simulink model "OMSv1_5_lfd"  (Simulink 7.0)
settings: Solver=ode4  SolverMode=SingleTasking  StartTime=0.0  StopTime=5  FixedStep=0.001  MaxStep=0.001  RelTol=1e-3  AbsTol=1e-3
undefined symbols (not defined in the file): alexlaw, bs_onoff, bs_scale, bsfsacrit, bsfsvcrit, cnsgain, fs_onoff, fs_scale, fsdelaycalc, ltdrk, mdlparamlist, phasicgain, pmcgain, pmctau2, pmctau3, saccsw, spgain, tonicgain, tvrD, tvrN
(part 2 of 11)

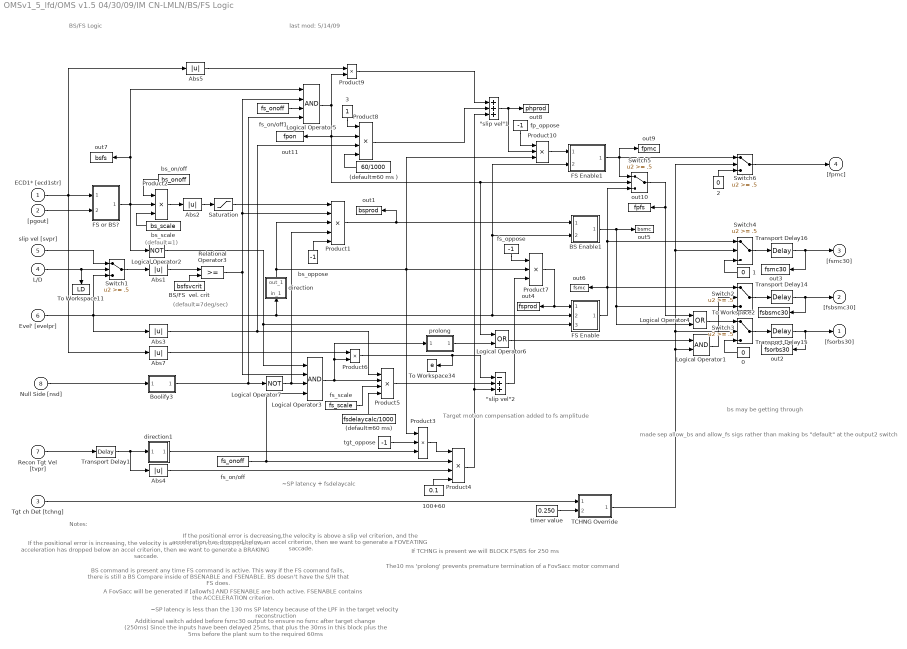
== system OMSv1_5_lfd/OMS v1.5 04/30/09/IM CN-LMLN/BS/FS Logic ==
  note: BS/FS Logic
  note: If the positional error is increasing, the velocity
      |  is above a slip vel criterion, and the acceleration
      | has dropped below an accel criterion, then we
      | want to generate a BRAKING saccade.
  note: If the positional error is decreasing,the velocity
      | is above a slip vel criterion, and the acceleration
      | has dropped below an accel criterion, then we
      | want to generate a FOVEATING saccade.
  note: last mod:
      | 5/14/09
  note: (default=7deg/sec)
  note: (default=1)
  note: If TCHNG is present we will BLOCK
      | FS/BS for 250 ms
  note: BS command is present any time FS command is active.  This way if the FS coomand fails, there is still a BS
      | Compare inside of BSENABLE and FSENABLE.  BS doesn't have the S/H that FS does.
  note: A FovSacc will be generated if [allowfs] AND FSENABLE are both active. FSENABLE contains the ACCELERATION criterion.
  note: Notes:
  note: The10 ms 'prolong' prevents premature
      | termination of a FovSacc motor command
  note: made sep allow_bs and allow_fs
      | sigs rather than making bs "default"
      | at the output2 switch
  note: bs may be getting through
  note: ~SP latency + fsdelaycalc
  note: Target motion compensation
      | added to fs amplitude
  note: ~SP latency is less than the 130 ms SP latency because of the LPF in the target velocity reconstruction
  note: Additional switch added before fsmc30 output to ensure no fsmc after target change (250ms)
      | Since the inputs have been delayed 25ms, that plus the 30ms in this block plus the 5ms before the plant sum to the required 60ms
  ECD1* [ecd1str] : Inport  OutDataType=sfix(16)  OutScaling=2^0
  "[pgout]" : Inport  Port=2  OutDataType=sfix(16)  OutScaling=2^0
  Tgt ch Det [tchng] : Inport  Port=3  OutDataType=sfix(16)  OutScaling=2^0
  L/D : Inport  Port=4  OutDataType=sfix(16)  OutScaling=2^0
  slip vel [svpr] : Inport  Port=5  OutDataType=sfix(16)  OutScaling=2^0
  Evel' [evelpr] : Inport  Port=6  OutDataType=sfix(16)  OutScaling=2^0
  Recon Tgt Vel [tvpr] : Inport  Port=7  OutDataType=sfix(16)  OutScaling=2^0
  Null Side [nsd] : Inport  Port=8  OutDataType=sfix(16)  OutScaling=2^0
  "\"slip vel\"1" : Sum  Inputs=+++  OutDataType=sfix(16)  OutScaling=2^0  SaturateOnIntegerOverflow=on  InputSameDT=on
  "\"slip vel\"2" : Sum  Inputs=-++  OutDataType=sfix(16)  OutScaling=2^0  SaturateOnIntegerOverflow=on  InputSameDT=on
  (default=60 ms ) : Constant  Orientation=left  Value=60/1000  OutDataType=sfix(16)  OutScaling=2^0
  (default=60 ms) : Constant  Orientation=up  Value=fsdelaycalc/1000  OutDataType=sfix(16)  OutScaling=2^0
  0 : Constant  Orientation=left  Value=0  OutDataType=sfix(16)  OutScaling=2^0
  1 : Constant  Orientation=left  Value=0  OutDataType=sfix(16)  OutScaling=2^0
  100+60 : Constant  Orientation=up  Value=0.1  OutDataType=sfix(16)  OutScaling=2^0
  2 : Constant  Orientation=up  Value=0  OutDataType=sfix(16)  OutScaling=2^0
  3 : Constant  Orientation=down  OutDataType=sfix(16)  OutScaling=2^0
  Abs{1..5,7} (6 alike) : Abs  SaturateOnIntegerOverflow=on
  BS Enable1 : Subsystem
      mask Display: disp('BS\nEnab')
  BS/FS  vel. crit : Constant  Orientation=up  Value=bsfsvcrit  OutDataType=sfix(16)  OutScaling=2^0
  Boolify3 : Subsystem
      mask Display: disp('Boolify')
  FS Enable : Subsystem
      mask Display: disp('FS\nEnab')
  FS Enable1 : Subsystem
      mask Display: disp('Fast Phase\nEnab')
  FS or BS? : Subsystem
      mask Display: disp('BS=1\nFS=0')
  Logical Operator1 : Logic
  Logical Operator2 : Logic  Operator=NOT  Inputs=1
  Logical Operator3 : Logic  Inputs=4
  Logical Operator4 : Logic  Operator=OR
  Logical Operator5 : Logic  Inputs=4
  Logical Operator6 : Logic  Operator=OR
  Logical Operator7 : Logic  Operator=NOT  Inputs=1
  Product1 : Product  Inputs=5  OutDataType=sfix(16)  OutScaling=2^0  SaturateOnIntegerOverflow=on  RndMeth=Zero  InputSameDT=on
  Product{2..3,7,10} (4 alike) : Product  Inputs=3  OutDataType=sfix(16)  OutScaling=2^0  SaturateOnIntegerOverflow=on  RndMeth=Zero  InputSameDT=on
  Product4 : Product  Inputs=4  OutDataType=sfix(16)  OutScaling=2^0  SaturateOnIntegerOverflow=on  RndMeth=Zero  InputSameDT=on
  Product5 : Product  Inputs=4  OutDataType=sfix(16)  OutScaling=2^0  SaturateOnIntegerOverflow=on  RndMeth=Zero  InputSameDT=on
  Product6 : Product  OutDataType=sfix(16)  OutScaling=2^0  SaturateOnIntegerOverflow=on  RndMeth=Zero  InputSameDT=on
  Product8 : Product  Inputs=4  OutDataType=sfix(16)  OutScaling=2^0  SaturateOnIntegerOverflow=on  RndMeth=Zero  InputSameDT=on
  Product9 : Product  OutDataType=sfix(16)  OutScaling=2^0  SaturateOnIntegerOverflow=on  RndMeth=Zero  InputSameDT=on
  Relational Operator3 : RelationalOperator  InputSameDT=on
  Saturation : Saturate  UpperLimit=2  LowerLimit=0
  Switch{1..6} (6 alike) : Switch  Threshold=.5  SaturateOnIntegerOverflow=on  InputSameDT=on
  TCHNG Override : Subsystem
      mask Display: disp('TCHNG\nOverride')
  To Workspace11 : ToWorkspace  VariableName=LD  SaveFormat=Array
      settings: Orientation=down  MaxDataPoints=10000
  To Workspace2 : ToWorkspace  VariableName=fsbsmc30  SaveFormat=Array
      settings: MaxDataPoints=10000
  To Workspace34 : ToWorkspace  VariableName=e  SaveFormat=Array
      settings: MaxDataPoints=10000
  Transport Delay1 : TransportDelay  DelayTime=0.05
      mask Display: disp('50ms')
  Transport Delay14 : TransportDelay  DelayTime=0.03
      mask Display: disp('30ms')
  Transport Delay15 : TransportDelay  DelayTime=0.03
      mask Display: disp('30ms')
  Transport Delay16 : TransportDelay  DelayTime=0.03
      mask Display: disp('30ms')
  bs_on/off : Constant  Orientation=left  Value=bs_onoff  OutDataType=sfix(16)  OutScaling=2^0
  bs_oppose : Constant  Orientation=up  Value=-1  OutDataType=sfix(16)  OutScaling=2^0
  bs_scale : Constant  Orientation=left  Value=bs_scale  OutDataType=sfix(16)  OutScaling=2^0
  direction : Subsystem  Orientation=up
      mask Type: Sign
      mask Description: y = sign(x)
      mask Help: Sign Function:\n\t\t\ty = 1 if x > 0\n\t\t\ty = 0 if x = 0\n\t\t\ty = -1 if x < 0
      mask Display: plot(-50,-50,50,50,[-50,50],[0,0],[0,0],[-50,50],[-40,0],[-30,-30],[0,40],[30,30])
  direction1 : Subsystem
      mask Type: Sign
      mask Description: y = sign(x)
      mask Help: Sign Function:\n\t\t\ty = 1 if x > 0\n\t\t\ty = 0 if x = 0\n\t\t\ty = -1 if x < 0
      mask Display: plot(-50,-50,50,50,[-50,50],[0,0],[0,0],[-50,50],[-40,0],[-30,-30],[0,40],[30,30])
  fp_oppose : Constant  Orientation=down  Value=-1  OutDataType=sfix(16)  OutScaling=2^0
  fs_on/off : Constant  Value=fs_onoff  OutDataType=sfix(16)  OutScaling=2^0
  fs_on/off1 : Constant  Value=fs_onoff  OutDataType=sfix(16)  OutScaling=2^0
  fs_oppose : Constant  Orientation=down  Value=-1  OutDataType=sfix(16)  OutScaling=2^0
  fs_scale : Constant  Value=fs_scale  OutDataType=sfix(16)  OutScaling=2^0
  out1 : ToWorkspace  VariableName=bsprod  SaveFormat=Array
      settings: MaxDataPoints=100000
  out10 : ToWorkspace  VariableName=fpfs  SaveFormat=Array
      settings: MaxDataPoints=100000
  out11 : ToWorkspace  VariableName=fpon  SaveFormat=Array
      settings: MaxDataPoints=100000
  out2 : ToWorkspace  VariableName=fsorbs30  SaveFormat=Array
      settings: MaxDataPoints=100000
  out3 : ToWorkspace  VariableName=fsmc30  SaveFormat=Array
      settings: MaxDataPoints=100000
  out4 : ToWorkspace  VariableName=fsprod  SaveFormat=Array
      settings: MaxDataPoints=100000
  out5 : ToWorkspace  VariableName=bsmc  SaveFormat=Array
      settings: MaxDataPoints=100000
  out6 : ToWorkspace  VariableName=fsmc  SaveFormat=Array
      settings: MaxDataPoints=100000
  out7 : ToWorkspace  VariableName=bsfs  SaveFormat=Array
      settings: MaxDataPoints=100000
  out8 : ToWorkspace  VariableName=phprod  SaveFormat=Array
      settings: MaxDataPoints=100000
  out9 : ToWorkspace  VariableName=fpmc  SaveFormat=Array
      settings: MaxDataPoints=100000
  prolong : Subsystem  mask{prolong=1}
      mask prompts: prolong "Prolong pulse by?  (msec)"
      mask Display: disp('prolong')
  tgt_oppose : Constant  Value=-1  OutDataType=sfix(16)  OutScaling=2^0
  timer value : Constant  Value=0.250  OutDataType=sfix(16)  OutScaling=2^0
  "[fsorbs30]" : Outport  OutDataType=sfix(16)  OutScaling=2^0  InitialOutput=0
  "[fsbsmc30]" : Outport  Port=2  OutDataType=sfix(16)  OutScaling=2^0  InitialOutput=0
  "[fsmc30]" : Outport  Port=3  OutDataType=sfix(16)  OutScaling=2^0  InitialOutput=0
  "[fpmc]" : Outport  Port=4  OutDataType=sfix(16)  OutScaling=2^0  InitialOutput=0
  wires:
  Abs2/1 -> Saturation/1
  FS or BS?/1(BS=1 FS=0) -> Product2/2, Logical Operator2/1, Logical Operator5/1, out7/1
  bs_on/off/1 -> Product2/1
  bs_scale/1 -> Product2/3
  slip vel [svpr]/1 -> Switch1/1
  Switch1/1 -> Abs1/1
  Evel' [evelpr]/1 -> Switch1/3, direction/1(in_1), FS Enable/2("[evelpr]"), BS Enable1/2("[evelpr]"), FS Enable1/2("[evelpr]"), Abs3/1
  Relational Operator3/1 -> Logical Operator3/2, Product1/2, Logical Operator5/2
  "[pgout]"/1 -> FS or BS?/2(pgout)
  ECD1* [ecd1str]/1 -> Abs5/1, FS or BS?/1(pos error [ecd1str]), Abs7/1
  BS/FS  vel. crit/1 -> Relational Operator3/2
  Abs1/1 -> Relational Operator3/1
  direction/1(out_1) -> Product1/3, Product7/2, Product10/3, Product3/1
  (default=60 ms)/1 -> Product5/4
  Abs3/1 -> Product5/1, Product8/3
  Logical Operator3/1 -> Product5/2, Product6/2, prolong/1(value(in))
  fs_oppose/1 -> Product7/1
  Abs7/1 -> Product6/1
  FS Enable/1("[fsmc]") -> Switch2/1, out6/1, Switch4/1, Switch5/3
  Switch2/1 -> Transport Delay14/1
  fs_scale/1 -> Product5/3
  Tgt ch Det [tchng]/1 -> TCHNG Override/1("[tchng]")
  timer value/1 -> TCHNG Override/2(timer dur)
  Transport Delay14/1 -> "[fsbsmc30]"/1, To Workspace2/1
  TCHNG Override/1(tchng sw) -> Switch4/2, Switch6/2, Switch3/2, Logical Operator1/2
  Transport Delay16/1 -> "[fsmc30]"/1, out3/1
  Product2/1 -> Abs2/1
  Saturation/1 -> Product1/1
  Product5/1 -> "\"slip vel\"2"/2
  Product7/1 -> FS Enable/1(fsprod), out4/1
  Product1/1 -> out1/1, BS Enable1/1(bsprod)
  BS Enable1/1("[bsmc]") -> out5/1, Switch2/3, Logical Operator4/2
  Logical Operator4/1 -> Switch3/1
  Switch3/1 -> Transport Delay15/1
  L/D/1 -> Switch1/2, To Workspace11/1
  Recon Tgt Vel [tvpr]/1 -> Transport Delay1/1
  Product3/1 -> Product4/1
  100+60/1 -> Product4/4
  direction1/1(out_1) -> Product3/3
  Abs4/1 -> Product4/3
  Product4/1 -> "\"slip vel\"2"/3, "\"slip vel\"1"/3
  "\"slip vel\"2"/1 -> Product7/3
  0/1 -> Switch3/3
  Logical Operator1/1 -> Switch2/2
  1/1 -> Switch4/3
  Switch4/1 -> Transport Delay16/1
  Transport Delay15/1 -> "[fsorbs30]"/1, out2/1
  Logical Operator2/1 -> Logical Operator3/1, FS Enable/3(fsbs?)
  Transport Delay1/1 -> direction1/1(in_1), Abs4/1
  Boolify3/1(Out1) -> Logical Operator7/1, Logical Operator5/4
  Null Side [nsd]/1 -> Boolify3/1(In1)
  fs_on/off/1 -> Product4/2, Logical Operator3/4
  Logical Operator7/1 -> Logical Operator3/3, Product1/4
  Logical Operator5/1 -> Product9/2, Product8/2, out11/1, Switch5/2, Logical Operator6/1
  (default=60 ms )/1 -> Product8/4
  Product8/1 -> "\"slip vel\"1"/2
  Product9/1 -> "\"slip vel\"1"/1
  "\"slip vel\"1"/1 -> out8/1, Product10/2
  fp_oppose/1 -> Product10/1
  Product10/1 -> FS Enable1/1(fsprod)
  FS Enable1/1("[fsmc]") -> Switch5/1, out9/1, Switch6/1
  2/1 -> Switch6/3
  Switch6/1 -> "[fpmc]"/1
  fs_on/off1/1 -> Logical Operator5/3
  Abs5/1 -> Product9/1
  3/1 -> Product8/1
  bs_oppose/1 -> Product1/5
  tgt_oppose/1 -> Product3/2
  Switch5/1 -> Logical Operator4/1, out10/1
  Logical Operator6/1 -> Logical Operator1/1
  Product6/1 -> "\"slip vel\"2"/1, To Workspace34/1
  prolong/1(value(out)) -> Logical Operator6/2

== system OMSv1_5_lfd/OMS v1.5 04/30/09/IM CN-LMLN/MdlPlnt+2 ==
  note: Plant Model+
  note: last mod:
      | 06/13/07
  note: fast
  note: slow
  "[eposspf]" : Inport  OutDataType=sfix(16)  OutScaling=2^0
  "[pgout]" : Inport  Port=2  OutDataType=sfix(16)  OutScaling=2^0
  "[epossps]" : Inport  Port=3  OutDataType=sfix(16)  OutScaling=2^0
  Derivative : Derivative
      mask Display: disp('s')
  NI Real2 : Subsystem
      mask Display: disp('Plant')
  OMN1 : Subsystem
      mask Display: disp('Slow\nOMN')
  OMN3 : Subsystem
      mask Display: disp('Fast\nOMN')
  To Workspace13 : ToWorkspace  VariableName=ecpy80  SaveFormat=Array
      settings: MaxDataPoints=10000
  To Workspace28 : ToWorkspace  VariableName=imvel  SaveFormat=Array
      settings: Orientation=down  MaxDataPoints=10000
      mask Type: imsw1in
  Transport Delay1 : TransportDelay  DelayTime=0.005
      mask Display: disp('5ms')
  Transport Delay12 : TransportDelay  DelayTime=0.075
      mask Display: disp('75ms')
  Transport Delay2 : TransportDelay  DelayTime=0.075
      mask Display: disp('75ms')
  Transport Delay3 : TransportDelay  DelayTime=0.005
      mask Display: disp('5ms')
  "[ecpy80]" : Outport  OutDataType=sfix(16)  OutScaling=2^0  InitialOutput=0
  "[imvel]" : Outport  Port=2  OutDataType=sfix(16)  OutScaling=2^0  InitialOutput=0
  wires:
  Derivative/1 -> Transport Delay2/1
  Transport Delay12/1 -> "[ecpy80]"/1, To Workspace13/1
  OMN3/1("[psout]") -> Transport Delay3/1
  Transport Delay1/1 -> NI Real2/2(slow components)
  OMN1/1("[psout]") -> Transport Delay1/1
  Transport Delay3/1 -> NI Real2/1(fast components)
  NI Real2/1(ecpyy) -> Derivative/1, Transport Delay12/1
  "[pgout]"/1 -> OMN3/2("[pgout]")
  "[eposspf]"/1 -> OMN3/1("[epossp]")
  Transport Delay2/1 -> "[imvel]"/1, To Workspace28/1
  "[epossps]"/1 -> OMN1/1("[epossp]")

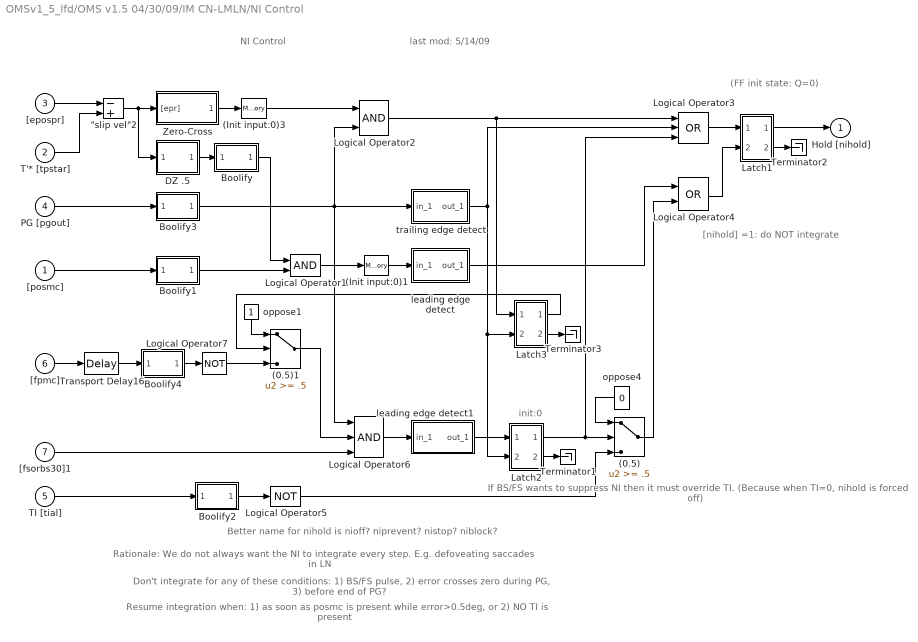
== system OMSv1_5_lfd/OMS v1.5 04/30/09/IM CN-LMLN/NI Control ==
  note: (FF init state: Q=0)
  note: NI Control
  note: If BS/FS wants to suppress NI
      | then it must override TI. (Because
      | when TI=0, nihold is forced off)
  note: last mod:
      | 5/14/09
  note: Rationale: We do not always want the NI to integrate every step. E.g. defoveating saccades in LN
  note: Don't integrate for any of these conditions: 1) BS/FS pulse, 2) error crosses zero during PG, 3) before end of PG?
  note: [nihold] =1: do NOT integrate
  note: init:0
  note: Better name for nihold is nioff? niprevent? nistop? niblock?
  note: Resume integration when: 1) as soon as posmc is present while error>0.5deg, or 2) NO TI is present
  "[posmc]" : Inport  OutDataType=sfix(16)  OutScaling=2^0
  T'* [tpstar] : Inport  Port=2  OutDataType=sfix(16)  OutScaling=2^0
  "[epospr]" : Inport  Port=3  OutDataType=sfix(16)  OutScaling=2^0
  PG [pgout] : Inport  Port=4  OutDataType=sfix(16)  OutScaling=2^0
  TI [tial] : Inport  Port=5  OutDataType=sfix(16)  OutScaling=2^0
  "[fpmc]" : Inport  Port=6  OutDataType=sfix(16)  OutScaling=2^0
  "[fsorbs30]1" : Inport  Port=7  OutDataType=sfix(16)  OutScaling=2^0
  "\"slip vel\"2" : Sum  Inputs=-+  OutDataType=sfix(16)  OutScaling=2^0  SaturateOnIntegerOverflow=on  InputSameDT=on
  (0.5) : Switch  Threshold=.5  SaturateOnIntegerOverflow=on  InputSameDT=on
  (0.5)1 : Switch  Threshold=.5  SaturateOnIntegerOverflow=on  InputSameDT=on
  (Init input:0)1 : Memory
  (Init input:0)3 : Memory
  Boolify : Subsystem
      mask Display: disp('Boolify')
  Boolify1 : Subsystem
      mask Display: disp('Boolify')
  Boolify2 : Subsystem
      mask Display: disp('Boolify')
  Boolify3 : Subsystem
      mask Display: disp('Boolify')
  Boolify4 : Subsystem
      mask Display: disp('Boolify')
  DZ .5 : Subsystem
      mask Display: disp('Dead\nZone')
  Latch1 : Subsystem  mask(Latch){@1=0}
      mask prompts: @1 "Initial State for Output "Q":"
      mask help: Latch
      mask init:
      | ini=(@1~=0);
      mask Help: Latches the S input.  When S (set) is one, the Q output  becomes one.  The output remains one until the R (reset) input becomes one, forcing the output to zero.  If both R and S are one, the latch will be in an undefined state.
      mask Display: disp('S   Q\n\nR  !Q')
  Latch2 : Subsystem  mask(Latch){@1=0}
      mask prompts: @1 "Initial State for Output "Q":"
      mask help: Latch
      mask init:
      | ini=(@1~=0);
      mask Help: Latches the S input.  When S (set) is one, the Q output  becomes one.  The output remains one until the R (reset) input becomes one, forcing the output to zero.  If both R and S are one, the latch will be in an undefined state.
      mask Display: disp('S   Q\n\nR  !Q')
  Latch3 : Subsystem  mask(Latch){@1=0}
      mask prompts: @1 "Initial State for Output "Q":"
      mask help: Latch
      mask init:
      | ini=(@1~=0);
      mask Help: Latches the S input.  When S (set) is one, the Q output  becomes one.  The output remains one until the R (reset) input becomes one, forcing the output to zero.  If both R and S are one, the latch will be in an undefined state.
      mask Display: disp('S   Q\n\nR  !Q')
  Logical Operator1 : Logic
  Logical Operator2 : Logic
  Logical Operator3 : Logic  Operator=OR  Inputs=3
  Logical Operator4 : Logic  Operator=OR
  Logical Operator5 : Logic  Operator=NOT  Inputs=1
  Logical Operator6 : Logic  Inputs=3
  Logical Operator7 : Logic  Operator=NOT  Inputs=1
  Terminator1 : Terminator
  Terminator2 : Terminator
  Terminator3 : Terminator
  Transport Delay16 : TransportDelay  DelayTime=0.03
      mask Display: disp('30ms')
  Zero-Cross : Subsystem
      mask Display: disp('Zero-Cross\nDetect')
  leading edge detect : Subsystem
      mask Display: disp('Leading\nEdge Det')
  leading edge detect1 : Subsystem
      mask Display: disp('Leading\nEdge Det')
  oppose1 : Constant  Orientation=down  OutDataType=sfix(16)  OutScaling=2^0
  oppose4 : Constant  Orientation=left  Value=0  OutDataType=sfix(16)  OutScaling=2^0
  trailing edge detect : Subsystem
      mask Display: disp('Trailing\nEdge Det')
  Hold [nihold] : Outport  OutDataType=sfix(16)  OutScaling=2^0  InitialOutput=0
  wires:
  T'* [tpstar]/1 -> "\"slip vel\"2"/2
  PG [pgout]/1 -> Boolify3/1(In1)
  "[epospr]"/1 -> "\"slip vel\"2"/1
  Latch1/1(out_1) -> Hold [nihold]/1
  Logical Operator1/1 -> (Init input:0)1/1
  oppose4/1 -> (0.5)/1
  Logical Operator5/1 -> (0.5)/3
  TI [tial]/1 -> Boolify2/1(In1)
  Boolify2/1(Out1) -> Logical Operator5/1
  (0.5)/1 -> Logical Operator4/2
  Boolify3/1(Out1) -> Logical Operator6/1, trailing edge detect/1(in_1), Logical Operator2/2
  trailing edge detect/1(out_1) -> Logical Operator3/2, Latch2/2(in_2), Latch3/2(in_2)
  "[posmc]"/1 -> Boolify1/1(In1)
  "\"slip vel\"2"/1 -> DZ .5/1(in_1), Zero-Cross/1("[epr]")
  Logical Operator2/1 -> Logical Operator3/1, Latch3/1(in_1)
  Logical Operator3/1 -> Latch1/1(in_1)
  Logical Operator4/1 -> Latch1/2(in_2)
  leading edge detect/1(out_1) -> Logical Operator4/1
  Boolify/1(Out1) -> Logical Operator1/1
  DZ .5/1(out_1) -> Boolify/1(In1)
  Boolify1/1(Out1) -> Logical Operator1/2
  Logical Operator6/1 -> leading edge detect1/1(in_1)
  leading edge detect1/1(out_1) -> Latch2/1(in_1)
  Latch2/2(out_2) -> Terminator1/1
  Latch1/2(out_2) -> Terminator2/1
  Zero-Cross/1("[epneq]") -> (Init input:0)3/1
  (Init input:0)3/1 -> Logical Operator2/1
  (Init input:0)1/1 -> leading edge detect/1(in_1)
  "[fsorbs30]1"/1 -> Logical Operator6/3
  Latch3/2(out_2) -> Terminator3/1
  (0.5)1/1 -> Logical Operator6/2
  Latch3/1(out_1) -> (0.5)1/2
  oppose1/1 -> (0.5)1/1
  Transport Delay16/1 -> Boolify4/1(In1)
  Boolify4/1(Out1) -> Logical Operator7/1
  "[fpmc]"/1 -> Transport Delay16/1
  Logical Operator7/1 -> (0.5)1/3
  Latch2/1(out_1) -> (0.5)/2, Logical Operator3/3

== system OMSv1_5_lfd/OMS v1.5 04/30/09/IM CN-LMLN/Sacc Blank ==
  note: Saccade and Post-Saccadic Drift Blanking
  note: (FF init state: Q=1)
  note: "Is RetVel Err increaing?"
  note: really an "enable"
      | signal?
  note: last mod:
      | 02/03/00
  note: [sbsac]  is initially ENABLED, and is DISABLED by  the leading edge of a saccade
      |  (after an 80ms delay).  70 ms later the timer REENABLES [sbsac]
      | (Because of the 80ms delay, actual time of reenable is150 ms after end of PG)
  note: Lower SR latch is SET by [sbsac] going high.  The switch will now pass information
      | about the change in velocity error (whether it is decreasing or increasing).
      | If it is increasing, [sbsp] is 1, and the beginning of this increase sets the switch so
      | that [sbsp] = [sbsac].  If the error is decreasing, then [sbsp] = 0, and should stay 0
      |  for as long as [velerr] is decreasing ***and hasn't crossed zero***
  note: Rationale: We do not want the model to look at the slow phase information that immediately
      | follows a saccade.   We want to disable both the saccadic and SP systems appropriately.
  note: Saccadic:
  note: SP:
  note: (init: Q=0)
  note: "non-decreasing"
  PG [pgout] : Inport  OutDataType=sfix(16)  OutScaling=2^0
  RetVelErr [velerr] : Inport  Port=2  OutDataType=sfix(16)  OutScaling=2^0
  Abs1 : Abs  SaturateOnIntegerOverflow=on
  Latch1 : Subsystem  mask(Latch){@1=1}
      mask prompts: @1 "Initial State for Output "Q":"
      mask help: Latch
      mask init:
      | ini=(@1~=0);
      mask Help: Latches the S input.  When S (set) is one, the Q output  becomes one.  The output remains one until the R (reset) input becomes one, forcing the output to zero.  If both R and S are one, the latch will be in an undefined state.
      mask Display: disp('S   Q\n\nR  !Q')
  Latch2 : Subsystem  mask(Latch){@1=0}
      mask prompts: @1 "Initial State for Output "Q":"
      mask help: Latch
      mask init:
      | ini=(@1~=0);
      mask Help: Latches the S input.  When S (set) is one, the Q output  becomes one.  The output remains one until the R (reset) input becomes one, forcing the output to zero.  If both R and S are one, the latch will be in an undefined state.
      mask Display: disp('S   Q\n\nR  !Q')
  Relational Operator : RelationalOperator  InputSameDT=on
  Switch5 : Switch  Threshold=.5  SaturateOnIntegerOverflow=on  InputSameDT=on
  Terminator : Terminator
  Terminator1 : Terminator
  To Workspace10 : ToWorkspace  VariableName=sbred  SaveFormat=Array
      settings: MaxDataPoints=10000
  To Workspace16 : ToWorkspace  VariableName=sbsac  SaveFormat=Array
      settings: MaxDataPoints=10000
  To Workspace22 : ToWorkspace  VariableName=sbsp  SaveFormat=Array
      settings: MaxDataPoints=10000
  Transport Delay1 : TransportDelay  DelayTime=0.08
      mask Display: disp('80ms')
  event timer1 : Subsystem
      mask Display: disp('Event\nTimer2')
  leading edge detect : Subsystem
      mask Display: disp('Leading\nEdge Det')
  loop breaker : Memory
  rising edge detect : Subsystem  Orientation=left
      mask Display: disp('Rising\nEdge Det')
  rising edge detect1 : Subsystem
      mask Display: disp('Rising\nEdge Det')
  timer value : Constant  Orientation=left  Value=0.07  OutDataType=sfix(16)  OutScaling=2^0
  SacBlnk [sbsac] : Outport  OutDataType=sfix(16)  OutScaling=2^0  InitialOutput=0
  SP S/H [sbsp] : Outport  Port=2  OutDataType=sfix(16)  OutScaling=2^0  InitialOutput=0
  wires:
  leading edge detect/1(out_1) -> Latch1/2(in_2)
  event timer1/1(out_1) -> Latch1/1(in_1)
  loop breaker/1 -> Relational Operator/2
  Abs1/1 -> loop breaker/1, Relational Operator/1
  Relational Operator/1 -> rising edge detect/1(in_1), Switch5/1
  rising edge detect1/1(out_1) -> To Workspace10/1, Latch2/1(in_1)
  RetVelErr [velerr]/1 -> Abs1/1
  PG [pgout]/1 -> Transport Delay1/1
  Transport Delay1/1 -> leading edge detect/1(in_1), event timer1/1(_PG)
  timer value/1 -> event timer1/2(_timer value (port))
  Latch1/1(out_1) -> SacBlnk [sbsac]/1, rising edge detect1/1(in_1), Switch5/3, To Workspace16/1
  rising edge detect/1(out_1) -> Latch2/2(in_2)
  Latch2/1(out_1) -> Switch5/2
  Switch5/1 -> SP S/H [sbsp]/1, To Workspace22/1
  Latch2/2(out_2) -> Terminator/1
  Latch1/2(out_2) -> Terminator1/1

== system OMSv1_5_lfd/OMS v1.5 04/30/09/IM CN-LMLN/Saccade Enable ==
  note: Saccade Enable
  note: last mod:
      | 07/11/07
  note: rfbenctrl
  note: ecenctrl
  note: e'*DZ
  note: for LN: make this
      | (fsorbs OR fphsz)
  note: TIDZ
  Tgt ch Det [tchng] : Inport  OutDataType=sfix(16)  OutScaling=2^0
  "[ecdstrdz]" : Inport  Port=2  OutDataType=sfix(16)  OutScaling=2^0
  "[err50]" : Inport  Port=3  OutDataType=sfix(16)  OutScaling=2^0
  "[pgout]" : Inport  Port=4  OutDataType=sfix(16)  OutScaling=2^0
  "[edot50]" : Inport  Port=5  OutDataType=sfix(16)  OutScaling=2^0
  "[tial]" : Inport  Port=6  OutDataType=sfix(16)  OutScaling=2^0
  "[sbsac]" : Inport  Port=7  OutDataType=sfix(16)  OutScaling=2^0
  "[fsorbs30]" : Inport  Port=8  OutDataType=sfix(16)  OutScaling=2^0
  Enable Control : Subsystem
      mask Display: disp('Enable\nControl')
  LN FPh Gen : Subsystem
      mask Display: disp('DFFPh\nGen')
  Latch1 : Subsystem  mask(Latch){@1=0}
      mask prompts: @1 "Initial State for Output "Q":"
      mask help: Latch
      mask init:
      | ini=(@1~=0);
      mask Help: Latches the S input.  When S (set) is one, the Q output  becomes one.  The output remains one until the R (reset) input becomes one, forcing the output to zero.  If both R and S are one, the latch will be in an undefined state.
      mask Display: disp('S   Q\n\nR  !Q')
  Logical Operator2 : Logic  Operator=NOT  Inputs=1
  Logical Operator3 : Logic
  Ret FB sample : Subsystem
      mask Display: disp('Ret FB\nEnab &\nSample')
  Terminator : Terminator
      settings: Orientation=down
  To Workspace14 : ToWorkspace  VariableName=sacenab  SaveFormat=Array
      settings: MaxDataPoints=10000
      mask Type: imsw1in
  To Workspace21 : ToWorkspace  VariableName=fphsz  SaveFormat=Array
      settings: MaxDataPoints=10000
  To Workspace25 : ToWorkspace  VariableName=rfbspl  SaveFormat=Array
      settings: MaxDataPoints=10000
      mask Type: imsw1in
  To Workspace5 : ToWorkspace  VariableName=ecpyenab  SaveFormat=Array
      settings: MaxDataPoints=10000
      mask Type: imsw1in
  Transport Delay1 : TransportDelay  DelayTime=0.025
      mask Display: disp('25ms')
  Transport Delay3 : TransportDelay  DelayTime=0.025
      mask Display: disp('25ms')
  leading edge detect2 : Subsystem
      mask Display: disp('Leading\nEdge Det')
  prolong : Subsystem  mask{prolong=10}
      mask prompts: prolong "Prolong pulse by?  (msec)"
      mask Display: disp('prolong')
  trailing edge detect : Subsystem
      mask Display: disp('Trailing\nEdge Det')
  "[rfbspl]" : Outport  OutDataType=sfix(16)  OutScaling=2^0  InitialOutput=0
  FPh Size [fphsz] : Outport  Port=2  OutDataType=sfix(16)  OutScaling=2^0  InitialOutput=0
  "[sacenab]" : Outport  Port=3  OutDataType=sfix(16)  OutScaling=2^0  InitialOutput=0
  wires:
  "[pgout]"/1 -> Logical Operator3/1, trailing edge detect/1(PG)
  Logical Operator2/1 -> Logical Operator3/2
  "[ecdstrdz]"/1 -> Enable Control/1(e'*DZ [ecdstrdz])
  Tgt ch Det [tchng]/1 -> LN FPh Gen/4(TCD [tchng]), Enable Control/3(Tgt ch Det [tchng])
  "[sbsac]"/1 -> LN FPh Gen/7("[sbsac]")
  "[edot50]"/1 -> Transport Delay1/1
  Enable Control/1(ECPY EnTmng [ecpyenab]) -> LN FPh Gen/3("[ecpyenab]"), Ret FB sample/1("[ecpyenab]"), To Workspace5/1
  "[err50]"/1 -> Transport Delay3/1
  Enable Control/2(RetFB En&Spl) -> Ret FB sample/2("[rfbenctrl]")
  LN FPh Gen/2(TIDZ) -> Ret FB sample/5(TIDZ)
  Ret FB sample/2(RetFB Enable [sacenab]) -> prolong/1(value(in)), LN FPh Gen/1("[rfbenab]")
  "[fsorbs30]"/1 -> leading edge detect2/1(in_1)
  leading edge detect2/1(out_1) -> Latch1/1(in_1)
  Latch1/1(out_1) -> Logical Operator2/1
  trailing edge detect/1(Latch R) -> Latch1/2(in_2)
  Logical Operator3/1 -> Enable Control/2(VolPG ( [pgout] &NOT fs or bs))
  LN FPh Gen/1("[eedot]") -> Ret FB sample/4("[eedot]")
  Ret FB sample/1(RFB Spl [rfbspl]) -> "[rfbspl]"/1, To Workspace25/1
  LN FPh Gen/3(FPh Size [fphsz]) -> FPh Size [fphsz]/1, To Workspace21/1
  prolong/1(value(out)) -> "[sacenab]"/1, To Workspace14/1
  "[tial]"/1 -> LN FPh Gen/5("[tial]"), Enable Control/4("[tial]")
  Latch1/2(out_2) -> Terminator/1
  Transport Delay3/1 -> Ret FB sample/3("[err50]"), LN FPh Gen/2("[err50]")
  Transport Delay1/1 -> LN FPh Gen/6("[edot50]")

== system OMSv1_5_lfd/OMS v1.5 04/30/09/IM CN-LMLN/Saccade Motor Commmand ==
  note: last mod:
      | 12/8/09
  note: Saccadic Motor Command
  note: If TCHNG occurs, BLOCK
      | BS/FS (and already prog vs?)
      | for 150 msec
  note: If TCHNG occurs:
      | ALLOW vol sacc
  note: make sure that tchngOVR
      | lets _something_ pass,
      | since it operates switches
      | in two different locations...
  "[ecdstrdz]" : Inport  OutDataType=sfix(16)  OutScaling=2^0
  "[fphsz]" : Inport  Port=2  OutDataType=sfix(16)  OutScaling=2^0
  Tgt ch Det [tchng] : Inport  Port=3  OutDataType=sfix(16)  OutScaling=2^0
  "[sacenab]" : Inport  Port=4  OutDataType=sfix(16)  OutScaling=2^0
  "[tvel]" : Inport  Port=5  OutDataType=sfix(16)  OutScaling=2^0
  fsorbs30 : Inport  Port=6  OutDataType=sfix(16)  OutScaling=2^0
  fsbcmc30 : Inport  Port=7  OutDataType=sfix(16)  OutScaling=2^0
  fsmc30 : Inport  Port=8  OutDataType=sfix(16)  OutScaling=2^0
  "\"slip vel\"1" : Sum  OutDataType=sfix(16)  OutScaling=2^0  SaturateOnIntegerOverflow=on  InputSameDT=on
  (0.5) : Switch  Threshold=.5  SaturateOnIntegerOverflow=on  InputSameDT=on
  (Init input:0)1 : Memory
  0 : Constant  Orientation=left  Value=0  OutDataType=sfix(16)  OutScaling=2^0
  Product1 : Product  OutDataType=sfix(16)  OutScaling=2^0  SaturateOnIntegerOverflow=on  RndMeth=Zero  InputSameDT=on
  Switch3 : Switch  Threshold=.5  SaturateOnIntegerOverflow=on  InputSameDT=on
  TCHNG Override : Subsystem
      mask Display: disp('TCHNG\nOverride')
  To Workspace1 : ToWorkspace  VariableName=errc  SaveFormat=Array
      settings: MaxDataPoints=10000
  To Workspace2 : ToWorkspace  VariableName=sacenabp  SaveFormat=Array
      settings: MaxDataPoints=10000
  To Workspace6 : ToWorkspace  VariableName=posmc  SaveFormat=Array
      settings: MaxDataPoints=10000
  Voluntary Saccade Switch : Subsystem
      mask Display: disp('Vol\nSacc\nSw')
  Voluntary Saccade Switch1 : Subsystem
      mask Display: disp('Corective\nSacc\nInhibition')
  prolong5 : Subsystem  mask{prolong=5}
      mask prompts: prolong "Prolong pulse by?  (msec)"
      mask Display: disp('IF prolong')
  timer value : Constant  Orientation=left  Value=0.15  OutDataType=sfix(16)  OutScaling=2^0
  "[posmc]" : Outport  OutDataType=sfix(16)  OutScaling=2^0  InitialOutput=0
  wires:
  "[sacenab]"/1 -> prolong5/1(value(in))
  0/1 -> Switch3/3
  (0.5)/1 -> Switch3/1
  Voluntary Saccade Switch/2(sacenab/0) -> (0.5)/2
  Tgt ch Det [tchng]/1 -> TCHNG Override/1("[tchng]"), prolong5/2(value(in)1), Voluntary Saccade Switch1/3(tchng)
  timer value/1 -> TCHNG Override/2(timer dur)
  Voluntary Saccade Switch/1("[vsmc]") -> (0.5)/1
  TCHNG Override/1(tchng sw) -> Switch3/2
  Switch3/1 -> To Workspace6/1, (Init input:0)1/1
  (Init input:0)1/1 -> "[posmc]"/1
  Voluntary Saccade Switch1/1("[vsmc]") -> Product1/1
  fsmc30/1 -> Voluntary Saccade Switch1/2(fsmc)
  prolong5/1(value(out)) -> Voluntary Saccade Switch/2("[sacenab]"), To Workspace2/1
  "[ecdstrdz]"/1 -> Product1/2
  Product1/1 -> "\"slip vel\"1"/1
  "[fphsz]"/1 -> "\"slip vel\"1"/2
  "\"slip vel\"1"/1 -> Voluntary Saccade Switch/1("[fphmag]"), To Workspace1/1
  "[tvel]"/1 -> Voluntary Saccade Switch1/1(tvel)
  fsbcmc30/1 -> (0.5)/3
  fsorbs30/1 -> Voluntary Saccade Switch/3("[fsorbs30]")

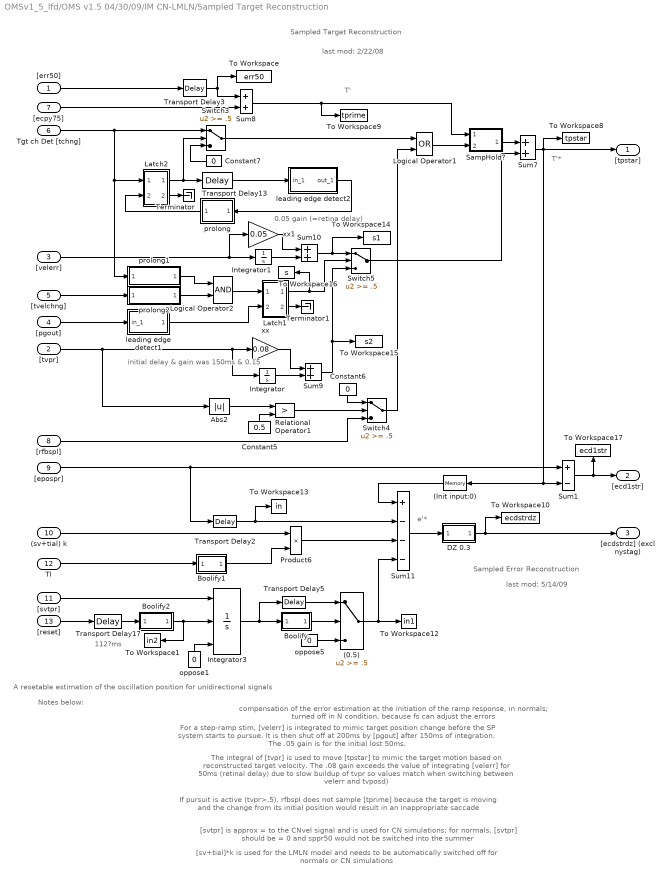
== system OMSv1_5_lfd/OMS v1.5 04/30/09/IM CN-LMLN/Sampled Target Reconstruction ==
  note: T'
  note: T'*
  note: Sampled Target Reconstruction
  note: last mod:
      | 2/22/08
  note: Notes below:
  note: If pursuit is active (tvpr>.5), rfbspl does not sample [tprime] because the target is moving and
      | the change from its initial position would result in an inappropriate saccade
  note: The integral of [tvpr] is used to move [tpstar] to mimic the target motion based on reconstructed target velocity. The .08 gain
      | exceeds the value of integrating [velerr] for 50ms (retinal delay) due to slow buildup of tvpr so values match
      | when switching between velerr and tvposd)
  note: For a step-ramp stim, [velerr] is integrated to mimic target position change before the SP system starts to pursue.
      |  It is then shut off at 200ms by [pgout] after 150ms of integration. The .05 gain is for the initial lost 50ms.
  note: initial delay & gain
      | was 150ms & 0.15
  note: 0.05 gain (=retina delay)
  note: e'*
  note: Sampled Error Reconstruction
  note: last mod:
      | 5/14/09
  note: [svtpr] is approx = to the CNvel signal and is used for CN simulations; for normals, [svtpr]
      | should be = 0 and sppr50 would not be switched into the summer
  note: [sv+tial]*k is used for the LMLN model and needs to be automatically switched off
      | for normals or CN simulations
  note: compensation of the error estimation at the initiation of the ramp response, in normals; turned off in N condition, because fs can adjust the errors
  note: 112?ms
  note: A resetable estimation of the oscillation position
      | for unidirectional signals
  "[err50]" : Inport  OutDataType=sfix(16)  OutScaling=2^0
  "[tvpr]" : Inport  Port=2  OutDataType=sfix(16)  OutScaling=2^0
  "[velerr]" : Inport  Port=3  OutDataType=sfix(16)  OutScaling=2^0
  "[pgout]" : Inport  Port=4  OutDataType=sfix(16)  OutScaling=2^0
  "[tvelchng]" : Inport  Port=5  OutDataType=sfix(16)  OutScaling=2^0
  Tgt ch Det [tchng] : Inport  Port=6  OutDataType=sfix(16)  OutScaling=2^0
  "[ecpy75]" : Inport  Port=7  OutDataType=sfix(16)  OutScaling=2^0
  "[rfbspl]" : Inport  Port=8  OutDataType=sfix(16)  OutScaling=2^0
  "[epospr]" : Inport  Port=9  OutDataType=sfix(16)  OutScaling=2^0
  (sv+tial) k : Inport  Port=10  OutDataType=sfix(16)  OutScaling=2^0
  "[svtpr]" : Inport  Port=11  OutDataType=sfix(16)  OutScaling=2^0
  TI : Inport  Port=12  OutDataType=sfix(16)  OutScaling=2^0
  "[reset]" : Inport  Port=13  OutDataType=sfix(16)  OutScaling=2^0
  (0.5) : Switch  Threshold=.5  SaturateOnIntegerOverflow=on  InputSameDT=on
  (Init input:0) : Memory  Orientation=left
  Abs2 : Abs  SaturateOnIntegerOverflow=on
  Boolify : Subsystem
      mask Display: disp('Boolify')
  Boolify1 : Subsystem
      mask Display: disp('Boolify')
  Boolify2 : Subsystem
      mask Display: disp('Boolify')
  Constant5 : Constant  Orientation=up  Value=0.5  OutDataType=sfix(16)  OutScaling=2^0
  Constant6 : Constant  Orientation=down  Value=0  OutDataType=sfix(16)  OutScaling=2^0
  Constant7 : Constant  Orientation=left  Value=0  OutDataType=sfix(16)  OutScaling=2^0
  DZ 0.3 : Subsystem
      mask Display: disp('DZ 0.3')
  Integrator : Integrator
  Integrator1 : Integrator
  Integrator3 : Integrator  ExternalReset=level  InitialConditionSource=external
  Latch1 : Subsystem  mask(Latch){@1=0}
      mask prompts: @1 "Initial State for Output "Q":"
      mask help: Latch
      mask init:
      | ini=(@1~=0);
      mask Help: Latches the S input.  When S (set) is one, the Q output  becomes one.  The output remains one until the R (reset) input becomes one, forcing the output to zero.  If both R and S are one, the latch will be in an undefined state.
      mask Display: disp('S   Q\n\nR  !Q')
  Latch2 : Subsystem  mask(Latch){@1=0}
      mask prompts: @1 "Initial State for Output "Q":"
      mask help: Latch
      mask init:
      | ini=(@1~=0);
      mask Help: Latches the S input.  When S (set) is one, the Q output  becomes one.  The output remains one until the R (reset) input becomes one, forcing the output to zero.  If both R and S are one, the latch will be in an undefined state.
      mask Display: disp('S   Q\n\nR  !Q')
  Logical Operator1 : Logic  Operator=OR
  Logical Operator2 : Logic
  Product6 : Product  OutDataType=sfix(16)  OutScaling=2^0  SaturateOnIntegerOverflow=on  RndMeth=Zero  InputSameDT=on
  Relational Operator1 : RelationalOperator  Operator=>  InputSameDT=on
  SampHold? : Subsystem
      mask Display: disp('S=H\nH=L')
  Sum1 : Sum  Inputs=+-  OutDataType=sfix(16)  OutScaling=2^0  SaturateOnIntegerOverflow=on  InputSameDT=on
  Sum{7..10} (4 alike) : Sum  OutDataType=sfix(16)  OutScaling=2^0  SaturateOnIntegerOverflow=on  InputSameDT=on
  Sum11 : Sum  Inputs=+---  OutDataType=sfix(16)  OutScaling=2^0  SaturateOnIntegerOverflow=on  InputSameDT=on
  Switch3 : Switch  Threshold=.5  SaturateOnIntegerOverflow=on  InputSameDT=on
  Switch4 : Switch  Threshold=.5  SaturateOnIntegerOverflow=on  InputSameDT=on
  Switch5 : Switch  Threshold=.5  SaturateOnIntegerOverflow=on  InputSameDT=on
  Terminator : Terminator
  Terminator1 : Terminator
  To Workspace : ToWorkspace  VariableName=err50  SaveFormat=Array
      settings: MaxDataPoints=10000
  To Workspace1 : ToWorkspace  VariableName=in2  SaveFormat=Array
      settings: MaxDataPoints=10000
  To Workspace10 : ToWorkspace  VariableName=ecdstrdz  SaveFormat=Array
      settings: MaxDataPoints=10000
  To Workspace12 : ToWorkspace  VariableName=in1  SaveFormat=Array
      settings: MaxDataPoints=10000
  To Workspace13 : ToWorkspace  VariableName=in  SaveFormat=Array
      settings: MaxDataPoints=10000
  To Workspace14 : ToWorkspace  VariableName=s1  SaveFormat=Array
      settings: MaxDataPoints=10000
  To Workspace15 : ToWorkspace  VariableName=s2  SaveFormat=Array
      settings: MaxDataPoints=10000
  To Workspace16 : ToWorkspace  VariableName=s  SaveFormat=Array
      settings: MaxDataPoints=10000
  To Workspace17 : ToWorkspace  VariableName=ecd1str  SaveFormat=Array
      settings: Orientation=up  MaxDataPoints=10000
  To Workspace8 : ToWorkspace  VariableName=tpstar  SaveFormat=Array
      settings: MaxDataPoints=10000
  To Workspace9 : ToWorkspace  VariableName=tprime  SaveFormat=Array
      settings: MaxDataPoints=10000
  Transport Delay13 : TransportDelay  DelayTime=0.05
      mask Display: disp('50ms')
  Transport Delay17 : TransportDelay  DelayTime=0.112
      mask Display: disp('delay')
  Transport Delay2 : TransportDelay  DelayTime=.075
      mask Display: disp('75ms')
  Transport Delay3 : TransportDelay  DelayTime=0.025
      mask Display: disp('25ms')
  Transport Delay5 : TransportDelay  DelayTime=.075  TransDelayFeedthrough=on
      mask Display: disp('75ms')
  leading edge detect1 : Subsystem
      mask Display: disp('Leading\nEdge Det')
  leading edge detect2 : Subsystem
      mask Display: disp('Leading\nEdge Det')
  oppose1 : Constant  Orientation=up  Value=0  OutDataType=sfix(16)  OutScaling=2^0
  oppose5 : Constant  Value=0  OutDataType=sfix(16)  OutScaling=2^0
  prolong : Subsystem  Orientation=left  mask{prolong=150}
      mask prompts: prolong "Prolong pulse by?  (msec)"
      mask Display: disp('150ms\nprolong')
  prolong1 : Subsystem  mask{prolong=5}
      mask prompts: prolong "Prolong pulse by?  (msec)"
      mask Display: disp('5ms prolong')
  prolong2 : Subsystem  mask{prolong=5}
      mask prompts: prolong "Prolong pulse by?  (msec)"
      mask Display: disp('5ms prolong')
  xx : Gain  Gain=0.08  ParameterDataType=sfix(16)  ParameterScaling=2^0  OutDataType=sfix(16)  OutScaling=2^0  SaturateOnIntegerOverflow=on
  xx1 : Gain  Gain=0.05  ParameterDataType=sfix(16)  ParameterScaling=2^0  OutDataType=sfix(16)  OutScaling=2^0  SaturateOnIntegerOverflow=on
  "[tpstar]" : Outport  OutDataType=sfix(16)  OutScaling=2^0  InitialOutput=0
  "[ecd1str]" : Outport  Port=2  OutDataType=sfix(16)  OutScaling=2^0  InitialOutput=0
  "[ecdstrdz] (excl nystag)" : Outport  Port=3  OutDataType=sfix(16)  OutScaling=2^0  InitialOutput=0
  wires:
  Sum8/1 -> To Workspace9/1, SampHold?/1(Input)
  "[ecpy75]"/1 -> Sum8/2
  prolong1/1(value(out)) -> Logical Operator2/1
  Tgt ch Det [tchng]/1 -> Latch2/1(in_1), prolong1/1(value(in)), Switch3/1
  Logical Operator1/1 -> SampHold?/2(S/H?)
  Sum7/1 -> "[tpstar]"/1, To Workspace8/1, (Init input:0)/1, Sum1/2
  SampHold?/1(output) -> Sum7/1
  Switch3/1 -> Logical Operator1/1
  Constant7/1 -> Switch3/3
  Latch2/1(out_1) -> Transport Delay13/1, Switch3/2
  Transport Delay13/1 -> leading edge detect2/1(in_1)
  leading edge detect2/1(out_1) -> prolong/1(value(in))
  prolong/1(value(out)) -> Latch2/2(in_2)
  Sum10/1 -> Switch5/1, To Workspace14/1
  Integrator1/1 -> Sum10/2
  xx1/1 -> Sum10/1
  Abs2/1 -> Relational Operator1/1
  Constant6/1 -> Switch4/1
  Constant5/1 -> Relational Operator1/2
  Relational Operator1/1 -> Switch4/2
  "[rfbspl]"/1 -> Switch4/3
  Integrator/1 -> Sum9/2
  xx/1 -> Sum9/1
  "[tvpr]"/1 -> Abs2/1, Integrator/1, xx/1
  Switch4/1 -> Logical Operator1/2
  leading edge detect1/1(out_1) -> Latch1/2(in_2)
  "[pgout]"/1 -> leading edge detect1/1(in_1)
  Logical Operator2/1 -> Latch1/1(in_1)
  prolong2/1(value(out)) -> Logical Operator2/2
  "[velerr]"/1 -> Integrator1/1, xx1/1
  Switch5/1 -> Sum7/2
  Latch1/1(out_1) -> Switch5/2, To Workspace16/1
  Sum9/1 -> Switch5/3, To Workspace15/1
  "[epospr]"/1 -> Transport Delay2/1, Sum1/1
  "[tvelchng]"/1 -> prolong2/1(value(in))
  Sum1/1 -> To Workspace17/1, "[ecd1str]"/1
  "[err50]"/1 -> Transport Delay3/1
  TI/1 -> Boolify1/1(In1)
  Boolify1/1(Out1) -> Product6/2
  (sv+tial) k/1 -> Product6/1
  Product6/1 -> Sum11/3
  oppose5/1 -> (0.5)/3
  "[svtpr]"/1 -> Integrator3/1
  Boolify/1(Out1) -> (0.5)/2
  (0.5)/1 -> Sum11/4, To Workspace12/1
  DZ 0.3/1(out_1) -> "[ecdstrdz] (excl nystag)"/1, To Workspace10/1
  Latch2/2(out_2) -> Terminator/1
  Latch1/2(out_2) -> Terminator1/1
  Transport Delay3/1 -> Sum8/1, To Workspace/1
  (Init input:0)/1 -> Sum11/1
  Transport Delay2/1 -> To Workspace13/1, Sum11/2
  Sum11/1 -> DZ 0.3/1(in_1)
  Transport Delay17/1 -> Boolify2/1(In1)
  "[reset]"/1 -> Transport Delay17/1
  oppose1/1 -> Integrator3/3
  Boolify2/1(Out1) -> Integrator3/2, To Workspace1/1
  Integrator3/1 -> Boolify/1(In1), Transport Delay5/1
  Transport Delay5/1 -> (0.5)/1

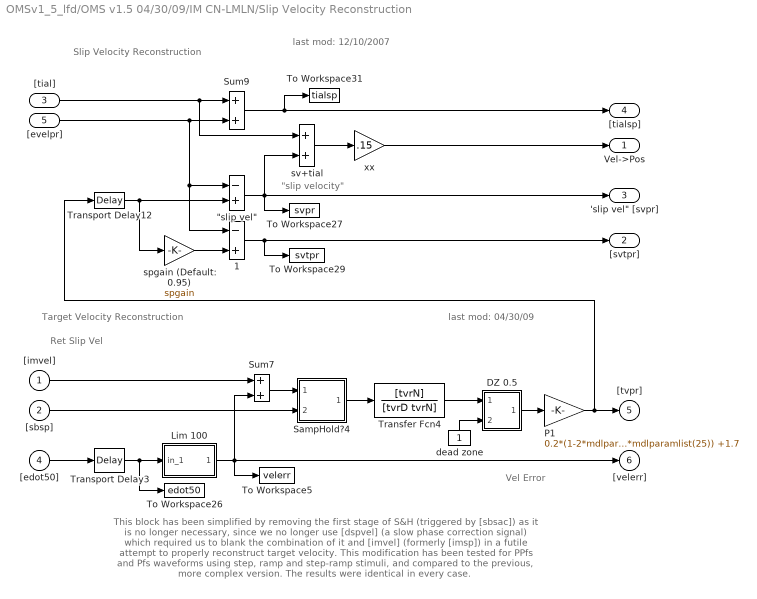
== system OMSv1_5_lfd/OMS v1.5 04/30/09/IM CN-LMLN/Slip Velocity Reconstruction ==
  note: last mod:
      | 12/10/2007
  note: Slip Velocity Reconstruction
  note: last mod:
      | 04/30/09
  note: Target Velocity Reconstruction
  note: This block has been simplified by removing the first stage of S&H (triggered by [sbsac]) as it is no longer necessary,
      | since we no longer use [dspvel] (a slow phase correction signal) which required us to blank the combination of it
      | and [imvel] (formerly [imsp]) in a futile attempt to properly reconstruct target velocity.  This modification has been tested
      | for PPfs and Pfs waveforms using step, ramp and step-ramp stimuli, and compared to the previous, more complex
      | version.  The results were identical in every case.
  note: "slip velocity"
  note: Vel
      | Error
  note: Ret Slip Vel
  "[imvel]" : Inport  OutDataType=sfix(16)  OutScaling=2^0
  "[sbsp]" : Inport  Port=2  OutDataType=sfix(16)  OutScaling=2^0
  "[tial]" : Inport  Port=3  OutDataType=sfix(16)  OutScaling=2^0
  "[edot50]" : Inport  Port=4  OutDataType=sfix(16)  OutScaling=2^0
  "[evelpr]" : Inport  Port=5  OutDataType=sfix(16)  OutScaling=2^0
  " 1" : Sum  Inputs=-+  OutDataType=sfix(16)  OutScaling=2^0  SaturateOnIntegerOverflow=on  InputSameDT=on
  "\"slip vel\"" : Sum  Inputs=-+  OutDataType=sfix(16)  OutScaling=2^0  SaturateOnIntegerOverflow=on  InputSameDT=on
  DZ 0.5 : Subsystem
      mask Display: disp('Dead\nZone')
  Lim 100 : Subsystem
      mask Display: disp('Limiter')
  P1 : Gain  Gain=0.2*(1-2*mdlparamlist(25))^2 -0.9*(1-2*mdlparamlist(25)) +1.7  ParameterDataType=sfix(16)  ParameterScaling=2^0  OutDataType=sfix(16)  OutScaling=2^0  SaturateOnIntegerOverflow=on
  SampHold?4 : Subsystem
      mask Display: disp('S=H\nH=L')
  Sum7 : Sum  OutDataType=sfix(16)  OutScaling=2^0  SaturateOnIntegerOverflow=on  InputSameDT=on
  Sum9 : Sum  OutDataType=sfix(16)  OutScaling=2^0  SaturateOnIntegerOverflow=on  InputSameDT=on
  To Workspace26 : ToWorkspace  VariableName=edot50  SaveFormat=Array
      settings: MaxDataPoints=10000
  To Workspace27 : ToWorkspace  VariableName=svpr  SaveFormat=Array
      settings: MaxDataPoints=10000
  To Workspace29 : ToWorkspace  VariableName=svtpr  SaveFormat=Array
      settings: MaxDataPoints=10000
  To Workspace31 : ToWorkspace  VariableName=tialsp  SaveFormat=Array
      settings: MaxDataPoints=10000
  To Workspace5 : ToWorkspace  VariableName=velerr  SaveFormat=Array
      settings: MaxDataPoints=10000
  Transfer Fcn4 : TransferFcn  Numerator=[tvrN]  Denominator=[tvrD tvrN]
  Transport Delay12 : TransportDelay  DelayTime=.05
      mask Display: disp('50ms')
  Transport Delay3 : TransportDelay  DelayTime=0.025
      mask Display: disp('25ms')
  dead zone : Constant  Orientation=up  OutDataType=sfix(16)  OutScaling=2^0
  spgain (Default: 0.95) : Gain  Gain=spgain  ParameterDataType=sfix(16)  ParameterScaling=2^0  OutDataType=sfix(16)  OutScaling=2^0  SaturateOnIntegerOverflow=on
  sv+tial : Sum  OutDataType=sfix(16)  OutScaling=2^0  SaturateOnIntegerOverflow=on  InputSameDT=on
  xx : Gain  Gain=.15  ParameterDataType=sfix(16)  ParameterScaling=2^0  OutDataType=sfix(16)  OutScaling=2^0  SaturateOnIntegerOverflow=on
  Vel->Pos : Outport  OutDataType=sfix(16)  OutScaling=2^0  InitialOutput=0
  "[svtpr]" : Outport  Port=2  OutDataType=sfix(16)  OutScaling=2^0  InitialOutput=0
  "'slip vel\" [svpr]" : Outport  Port=3  OutDataType=sfix(16)  OutScaling=2^0  InitialOutput=0
  "[tialsp]" : Outport  Port=4  OutDataType=sfix(16)  OutScaling=2^0  InitialOutput=0
  "[tvpr]" : Outport  Port=5  OutDataType=sfix(16)  OutScaling=2^0  InitialOutput=0
  "[velerr]" : Outport  Port=6  OutDataType=sfix(16)  OutScaling=2^0  InitialOutput=0
  wires:
  xx/1 -> Vel->Pos/1
  sv+tial/1 -> xx/1
  "[tial]"/1 -> sv+tial/1, Sum9/1
  "\"slip vel\""/1 -> sv+tial/2, To Workspace27/1, "'slip vel\" [svpr]"/1
  "[evelpr]"/1 -> Sum9/2, "\"slip vel\""/1, " 1"/1
  spgain (Default: 0.95)/1 -> " 1"/2
  " 1"/1 -> "[svtpr]"/1, To Workspace29/1
  Transport Delay12/1 -> "\"slip vel\""/2, spgain (Default: 0.95)/1
  dead zone/1 -> DZ 0.5/2(in_2)
  DZ 0.5/1(out_1) -> P1/1
  "[sbsp]"/1 -> SampHold?4/2(S/H?)
  Lim 100/1(out_1) -> "[velerr]"/1, To Workspace5/1, Sum7/2
  Sum7/1 -> SampHold?4/1(Input)
  SampHold?4/1(output) -> Transfer Fcn4/1
  Transfer Fcn4/1 -> DZ 0.5/1(in_1)
  Sum9/1 -> To Workspace31/1, "[tialsp]"/1
  "[edot50]"/1 -> Transport Delay3/1
  P1/1 -> "[tvpr]"/1, Transport Delay12/1
  Transport Delay3/1 -> Lim 100/1(in_1), To Workspace26/1
  "[imvel]"/1 -> Sum7/1

== system OMSv1_5_lfd/OMS v1.5 04/30/09/IM CN-LMLN/Target Change Detection ==
  note: Target Change Detection
  note: Detects T change >1 deg any time
  note: 12/10/07
  RetErr Vel [edot50] : Inport  OutDataType=sfix(16)  OutScaling=2^0
  "[tvpr]" : Inport  Port=2  OutDataType=sfix(16)  OutScaling=2^0
  Abs2 : Abs  SaturateOnIntegerOverflow=on
  Abs3 : Abs  SaturateOnIntegerOverflow=on
  Constant5 : Constant  Orientation=up  Value=950  OutDataType=sfix(16)  OutScaling=2^0
  Constant6 : Constant  Orientation=up  Value=950  OutDataType=sfix(16)  OutScaling=2^0
  Derivative : Derivative
      mask Display: disp('s')
  Relational Operator : RelationalOperator  InputSameDT=on
  Relational Operator1 : RelationalOperator  InputSameDT=on
  To Workspace20 : ToWorkspace  VariableName=tchng  SaveFormat=Array
      settings: MaxDataPoints=10000
  Transport Delay3 : TransportDelay  DelayTime=0.025
      mask Display: disp('25ms')
  Tvel Chng [tvelchng] : Outport  OutDataType=sfix(16)  OutScaling=2^0  InitialOutput=0
  Trgt Chng [tchng] : Outport  Port=2  OutDataType=sfix(16)  OutScaling=2^0  InitialOutput=0
  wires:
  RetErr Vel [edot50]/1 -> Abs2/1
  Constant5/1 -> Relational Operator/2
  Abs2/1 -> Relational Operator/1
  Constant6/1 -> Relational Operator1/2
  Abs3/1 -> Relational Operator1/1
  "[tvpr]"/1 -> Derivative/1
  Derivative/1 -> Abs3/1
  Relational Operator1/1 -> Tvel Chng [tvelchng]/1
  Relational Operator/1 -> To Workspace20/1, Transport Delay3/1
  Transport Delay3/1 -> Trgt Chng [tchng]/1

== system OMSv1_5_lfd/OMS v1.5 04/30/09/IM CN-LMLN/setmdlp ==

== system OMSv1_5_lfd/OMS v1.5 04/30/09/NI Real2/2-PPlntSat ==
  note: A 2-pole plant can be simulated by:
      | 1. no limitation on lateral gaze
      | 2. a hard limitation - placing a saturation in the plant [eg, 55 deg]
      | 3. a soft limitation - add the dead zone  [DZ slope>0]
  in_1 : Inport  OutDataType=sfix(16)  OutScaling=2^0
  2 pole : ZeroPole  Zeros=[ ]  Poles=[ -1/.18 -1/.007]  Gain=[1/.18 * 1/.007]
      mask Display: disp('2-pole\nPlant')
  DZ slope : Constant  Value=0.05  OutDataType=sfix(16)  OutScaling=2^0
  Dead Zone : DeadZone  LowerValue=-55  UpperValue=55  SaturateOnIntegerOverflow=on
  Product : Product  OutDataType=sfix(16)  OutScaling=2^0  SaturateOnIntegerOverflow=on  RndMeth=Zero  InputSameDT=on
  Saturation : Saturate  UpperLimit=55  LowerLimit=-55
  Sum3 : Sum  OutDataType=sfix(16)  OutScaling=2^0  SaturateOnIntegerOverflow=on  InputSameDT=on
  out_1 : Outport  OutDataType=sfix(16)  OutScaling=2^0  InitialOutput=0
  wires:
  DZ slope/1 -> Product/2
  Product/1 -> Sum3/2
  Sum3/1 -> out_1/1
  Saturation/1 -> Sum3/1
  Dead Zone/1 -> Product/1
  2 pole/1 -> Saturation/1, Dead Zone/1
  in_1/1 -> 2 pole/1

== system OMSv1_5_lfd/OMS v1.5 04/30/09/NI Real3/Boolify1 ==
  In1 : Inport  OutDataType=sfix(16)  OutScaling=2^0
  Abs2 : Abs  SaturateOnIntegerOverflow=on
  Switch2 : Switch  Threshold=0.1  SaturateOnIntegerOverflow=on  InputSameDT=on
  Threshold 5 : Constant  OutDataType=sfix(16)  OutScaling=2^0
  Threshold 6 : Constant  Value=0  OutDataType=sfix(16)  OutScaling=2^0
  Out1 : Outport  OutDataType=sfix(16)  OutScaling=2^0  InitialOutput=0
  wires:
  Threshold 5/1 -> Switch2/1
  Threshold 6/1 -> Switch2/3
  Switch2/1 -> Out1/1
  In1/1 -> Abs2/1
  Abs2/1 -> Switch2/2
